simulink model "Copy_of_model_test_old"  (R2018b)
settings: Solver=ode5  StartTime=0.0  StopTime=1  FixedStep=0.01  RelTol=1e-3
values from neighbouring files (symbols this model uses):
  g = 9.81    [equations.m]    (also in general.m; general_lqi.m)
  m = 0.06    [equations.m]    (also in general.m = 0.057; general_lqi.m = 0.057)
  R = 1    [evaluateL.m]    (also in general.m = 4; general_lqi.m = 4)
  u_0 = R*x3_0    [general.m]    (also in general_lqi.m)
  x1_0 = 0.01    [general.m]    (also in general_lqi.m)
  x2_0 = 0    [general.m]    (also in general_lqi.m)
  x3_0 = sqrt((-2*m*g)/first(x1_0))    [general.m]    (also in general_lqi.m)
settings Model: Creator=Kinga  LastModifiedBy=Kinga

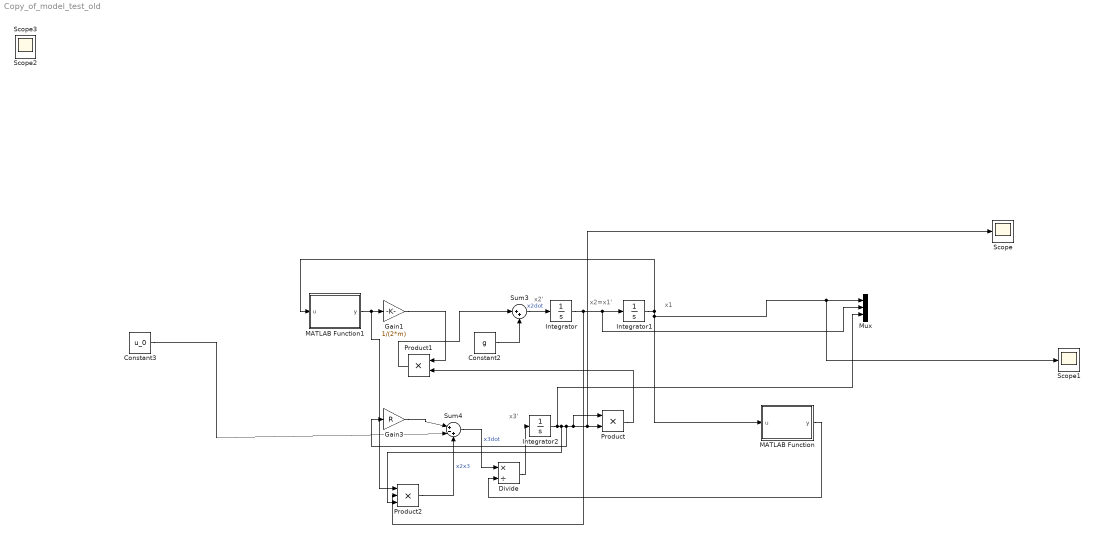
== system Copy_of_model_test_old ==
  note: x3'
  note: x1
  note: x2=x1'
  note: x2'
  Constant2 : Constant  Value=g
  Constant3 : Constant  Value=u_0
  Divide : Product  Inputs=*/
  Gain1 : Gain  Gain=1/(2*m)
  Gain3 : Gain  Gain=R
  Integrator : Integrator  InitialCondition=x2_0
  Integrator1 : Integrator  InitialCondition=x1_0
  Integrator2 : Integrator  InitialCondition=x3_0
  MATLAB Function : MATLAB Function  TreatAsAtomicUnit=on
  MATLAB Function1 : MATLAB Function  TreatAsAtomicUnit=on
  Mux : Mux  Inputs=3
  Product : Product
  Product1 : Product
  Product2 : Product  Inputs=3
  Scope{,1..3} (4 alike) : Scope
  Sum3 : Sum  Inputs=|++
  Sum4 : Sum  Inputs=|+-+
  wires:
  Sum3/1 -> Integrator/1  "x2dot"
  Constant2/1 -> Sum3/2
  Integrator/1 -> Product2/2, Mux/2, Integrator1/1
  MATLAB Function1/1(y) -> Product2/1, Gain1/1
  Integrator1/1 -> Scope1/1, Mux/1, MATLAB Function/1(u), MATLAB Function1/1(u)
  Product/1 -> Product1/2
  Gain1/1 -> Product1/1
  Product1/1 -> Sum3/1
  Gain3/1 -> Sum4/1
  Sum4/1 -> Divide/1  "x3dot"
  MATLAB Function/1(y) -> Divide/2
  Divide/1 -> Integrator2/1
  Product2/1 -> Sum4/3  "x2x3"
  Integrator2/1 -> Mux/3, Product2/3, Gain3/1, Product/1, Scope/1, Product/2
  Constant3/1 -> Sum4/2

== matlab function Copy_of_model_test_old/MATLAB Function1 ==
  data: u input; y output
function y = first(u)

a = 0.1017;
b = 0.01801;
c = -158.7;

y = c*b*exp(c*u);

== matlab function Copy_of_model_test_old/MATLAB Function ==
  data: u input; y output
function y = base(u)

a = 0.1017;
b = 0.01801;
c = -158.7;

y = a+b*exp(c*u);
